simulink model "chap5_3sim"  (R2016a)
settings: Solver=ode45  StartTime=0.0  StopTime=10.0  RelTol=1e-6
settings Model: Creator=zhanghankui  LastModifiedBy=zhanghankui

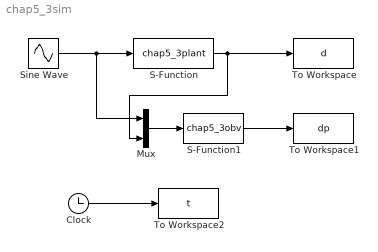
== system chap5_3sim ==
  Clock : Clock
  Mux : Mux  Inputs=2
  S-Function : S-Function  FunctionName=chap5_3plant  SFunctionDeploymentMode=off  EnableBusSupport=off
  S-Function1 : S-Function  FunctionName=chap5_3obv  SFunctionDeploymentMode=off  EnableBusSupport=off
  Sine Wave : Sin  SampleTime=0
  To Workspace : ToWorkspace  VariableName=d  SampleTime=-1
  To Workspace1 : ToWorkspace  VariableName=dp  SampleTime=-1
  To Workspace2 : ToWorkspace  VariableName=t  SampleTime=-1
  wires:
  Sine Wave/1 -> Mux/1, S-Function/1
  Mux/1 -> S-Function1/1
  S-Function/1 -> To Workspace/1, Mux/2
  S-Function1/1 -> To Workspace1/1
  Clock/1 -> To Workspace2/1
